simulink subsystem "MCD"  (R2023b)
settings: Solver=VariableStepAuto  StartTime=0.0  StopTime=10.0  RelTol=1e-3
settings Model: Creator=Usuario_UMA  LastModifiedBy=Usuario_UMA

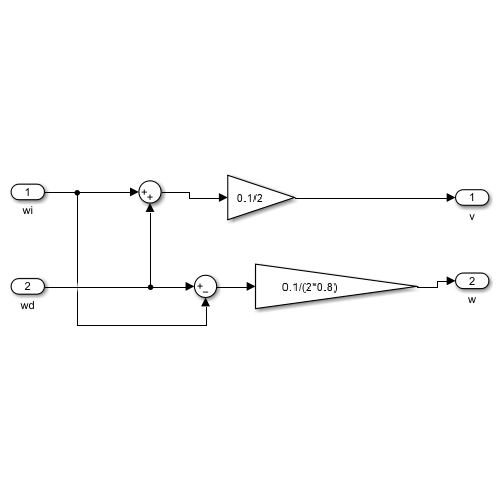
[thumbnail: Simulink's stored preview of the top-level diagram]
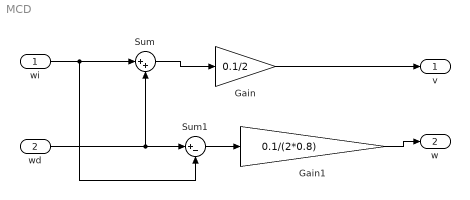
== system MCD ==
  wi : Inport
  wd : Inport  Port=2
  Gain : Gain  Gain=0.1/2
  Gain1 : Gain  Gain=0.1/(2*0.8)
  Sum : Sum  Inputs=|++
  Sum1 : Sum  Inputs=|+-
  v : Outport
  w : Outport  Port=2
  wires:
  wi/1 -> Sum1/2, Sum/1
  wd/1 -> Sum1/1, Sum/2
  Sum/1 -> Gain/1
  Gain/1 -> v/1
  Gain1/1 -> w/1
  Sum1/1 -> Gain1/1
